simulink model "IEEE_9bus_4"  (Simulink 8.4)
settings: Solver=ode4  StartTime=0.0  StopTime=inf  FixedStep=Ts  RelTol=1e-3
PostLoadFcn:
  | Ts=25e-6;Rs=5*1.867;cs=1.4080e-004;
InitFcn:
  | Ts=25e-6;Rs=5*1.867;cs=1.4080e-004;
undefined symbols (not defined in the file): another_event_name, gcbh, my_event_name, sps_rtmsupport
libraries: spsVIMeasurementModel x36, powerlib x34, powerlib_meascontrol x18, rtlab x4, artemis x3, sps_avr x3
(part 2 of 3)

== system IEEE_9bus_4/SM_System/Bus_4 230 KV ==
  Three-Phase V-I Measurement1 : Subsystem  DialogController=POWERSYS.PowerSysDialog  LoadFcn=sps_rtmsupport('LoadFcn',gcbh);  StartFcn=sps_rtmsupport('StartFcn',gcbh);  StopFcn=sps_rtmsupport('StopFcn',gcbh);  mask(Three-Phase VI Measurement){VoltageMeasurement=phase-to-phase, SetLabelV=on, LabelV=Vabc_4, Vpu=off, VpuLL=off, CurrentMeasurement=yes, SetLabelI=on, LabelI=Iabc_4, Ipu=off, Pbase=100e6, Vbase=230e3, OutputType=Complex, PhasorSimulation=off, PSBequivalent=0}
      mask prompts: VoltageMeasurement "Voltage measurement"; SetLabelV "Use a label"; LabelV "Signal label  (use a From block to collect this signal)"; Vpu "Voltages in pu,  based on peak value of nominal phase-to-ground voltage"; VpuLL "Voltages in pu,  based on peak value of nominal phase-to-phase  voltage"; CurrentMeasurement "Current measurement"; SetLabelI "Use a label"; LabelI "Signal label  (use a From block to collect this signal)"; Ipu "Currents in pu"; Pbase "Base power ( VA 3 phase)"; Vbase "Nominal voltage used for pu measurement (Vrms phase-phase) :"; OutputType "Output signals in:"; PhasorSimulation "Phasor simulation (internal use)"; PSBequivalent "Equivalent circuit (internal use)"
      mask help:
      | Ideal three-phase voltage and current measurements.
      |
      | The block can output the voltages and currents in per unit values or in volts and amperes.
      mask init: same as IEEE_9bus_4/SM_System/Bus_1 16.5 KV
      settings: CopyFcn=sps_rtmsupport('CopyFcn',gcbh); powericon('ThreePhaseVIMeasurementCopy',gcb)  DeleteFcn=sps_rtmsupport('DeleteFcn',gcbh);  UndoDeleteFcn=sps_rtmsupport('UndoDeleteFcn',gcbh);  ModelCloseFcn=sps_rtmsupport('ModelCloseFcn',gcbh);  PreSaveFcn="sps_rtmsupport('PreSaveFcn',gcbh);  set_param(gcb,'LinkStatus','restore')"  PostSaveFcn=sps_rtmsupport('PostSaveFcn',gcbh);  NameChangeFcn=sps_rtmsupport('NameChangeFcn',gcbh);  PreCopyFcn=sps_rtmsupport('PreCopyFcn',gcbh);  OpenFcn=sps_rtmsupport('OpenFcn',gcbh, [1 2 4 5 6 7 9 -12 13]);  CloseFcn=sps_rtmsupport('CloseFcn',gcbh);  PreDeleteFcn=sps_rtmsupport('PreDeleteFcn',gcbh);
      mask Help: helpview(psbhelp)
      mask TypeOptions VoltageMeasurement: no | phase-to-ground | phase-to-phase
      mask Callback VoltageMeasurement: powericon('ThreePhaseVIMeasurementCback',gcb,'Vselector');
      mask Callback SetLabelV: powericon('ThreePhaseVIMeasurementCback',gcb,'');
      mask Callback Vpu: powericon('ThreePhaseVIMeasurementCback',gcb,'Vpu');
      mask Callback VpuLL: powericon('ThreePhaseVIMeasurementCback',gcb,'VpuLL');
      mask TypeOptions CurrentMeasurement: no | yes
      mask Callback CurrentMeasurement: powericon('ThreePhaseVIMeasurementCback',gcb,'');
      mask Callback SetLabelI: powericon('ThreePhaseVIMeasurementCback',gcb,'');
      mask Callback LabelI: powericon('ThreePhaseVIMeasurementCback',gcb,'');
      mask Callback Ipu: powericon('ThreePhaseVIMeasurementCback',gcb,'');
      mask TypeOptions OutputType: Complex | Real-Imag | Magnitude-Angle | Magnitude
  Three-Phase V-I Measurement3 : Subsystem  DialogController=POWERSYS.PowerSysDialog  LoadFcn=sps_rtmsupport('LoadFcn',gcbh);  StartFcn=sps_rtmsupport('StartFcn',gcbh);  StopFcn=sps_rtmsupport('StopFcn',gcbh);  mask(Three-Phase VI Measurement){VoltageMeasurement=phase-to-phase, SetLabelV=on, LabelV=Vabc_46, Vpu=off, VpuLL=off, CurrentMeasurement=yes, SetLabelI=on, LabelI=Iabc_46, Ipu=off, Pbase=100e6, Vbase=230e3, OutputType=Complex, PhasorSimulation=off, PSBequivalent=0}
      mask prompts: VoltageMeasurement "Voltage measurement"; SetLabelV "Use a label"; LabelV "Signal label  (use a From block to collect this signal)"; Vpu "Voltages in pu,  based on peak value of nominal phase-to-ground voltage"; VpuLL "Voltages in pu,  based on peak value of nominal phase-to-phase  voltage"; CurrentMeasurement "Current measurement"; SetLabelI "Use a label"; LabelI "Signal label  (use a From block to collect this signal)"; Ipu "Currents in pu"; Pbase "Base power ( VA 3 phase)"; Vbase "Nominal voltage used for pu measurement (Vrms phase-phase) :"; OutputType "Output signals in:"; PhasorSimulation "Phasor simulation (internal use)"; PSBequivalent "Equivalent circuit (internal use)"
      mask help:
      | Ideal three-phase voltage and current measurements.
      |
      | The block can output the voltages and currents in per unit values or in volts and amperes.
      mask init: same as IEEE_9bus_4/SM_System/Bus_1 16.5 KV
      settings: CopyFcn=sps_rtmsupport('CopyFcn',gcbh); powericon('ThreePhaseVIMeasurementCopy',gcb)  DeleteFcn=sps_rtmsupport('DeleteFcn',gcbh);  UndoDeleteFcn=sps_rtmsupport('UndoDeleteFcn',gcbh);  ModelCloseFcn=sps_rtmsupport('ModelCloseFcn',gcbh);  PreSaveFcn="sps_rtmsupport('PreSaveFcn',gcbh);  set_param(gcb,'LinkStatus','restore')"  PostSaveFcn=sps_rtmsupport('PostSaveFcn',gcbh);  NameChangeFcn=sps_rtmsupport('NameChangeFcn',gcbh);  PreCopyFcn=sps_rtmsupport('PreCopyFcn',gcbh);  OpenFcn=sps_rtmsupport('OpenFcn',gcbh, [1 2 4 5 6 7 9 -12 13]);  CloseFcn=sps_rtmsupport('CloseFcn',gcbh);  PreDeleteFcn=sps_rtmsupport('PreDeleteFcn',gcbh);
      mask Help: helpview(psbhelp)
      mask TypeOptions VoltageMeasurement: no | phase-to-ground | phase-to-phase
      mask Callback VoltageMeasurement: powericon('ThreePhaseVIMeasurementCback',gcb,'Vselector');
      mask Callback SetLabelV: powericon('ThreePhaseVIMeasurementCback',gcb,'');
      mask Callback Vpu: powericon('ThreePhaseVIMeasurementCback',gcb,'Vpu');
      mask Callback VpuLL: powericon('ThreePhaseVIMeasurementCback',gcb,'VpuLL');
      mask TypeOptions CurrentMeasurement: no | yes
      mask Callback CurrentMeasurement: powericon('ThreePhaseVIMeasurementCback',gcb,'');
      mask Callback SetLabelI: powericon('ThreePhaseVIMeasurementCback',gcb,'');
      mask Callback LabelI: powericon('ThreePhaseVIMeasurementCback',gcb,'');
      mask Callback Ipu: powericon('ThreePhaseVIMeasurementCback',gcb,'');
      mask TypeOptions OutputType: Complex | Real-Imag | Magnitude-Angle | Magnitude
  Conn7 : PMIOPort  Port=1  Side=Left
  Conn8 : PMIOPort  Port=2  Side=Left
  Conn9 : PMIOPort  Port=3  Side=Left
  Conn1 : PMIOPort  Port=4  Side=Right
  Conn2 : PMIOPort  Port=5  Side=Right
  Conn3 : PMIOPort  Port=6  Side=Right
  Conn4 : PMIOPort  Port=7  Side=Right
  Conn5 : PMIOPort  Port=8  Side=Right
  Conn6 : PMIOPort  Port=9  Side=Right
  connections:
  Three-Phase V-I Measurement3/LConn3 -- Conn9/RConn1 -- Three-Phase V-I Measurement1/LConn3
  Three-Phase V-I Measurement3/LConn2 -- Conn8/RConn1 -- Three-Phase V-I Measurement1/LConn2
  Three-Phase V-I Measurement3/LConn1 -- Conn7/RConn1 -- Three-Phase V-I Measurement1/LConn1
  Three-Phase V-I Measurement3/RConn3 -- Conn6/RConn1
  Three-Phase V-I Measurement1/RConn3 -- Conn3/RConn1
  Three-Phase V-I Measurement1/RConn1 -- Conn1/RConn1
  Three-Phase V-I Measurement1/RConn2 -- Conn2/RConn1
  Three-Phase V-I Measurement3/RConn1 -- Conn4/RConn1
  Three-Phase V-I Measurement3/RConn2 -- Conn5/RConn1

== system IEEE_9bus_4/SM_System/Bus_5 230 KV ==
  Kv : Gain  Gain=Ki  SaturateOnIntegerOverflow=on  OutDataTypeStr=Inherit: Same as input  ParamDataTypeStr=Inherit: Same as input
  Kv1 : Gain  Gain=Kv  SaturateOnIntegerOverflow=on  OutDataTypeStr=Inherit: Same as input  ParamDataTypeStr=Inherit: Same as input
  Mode I : spsVIMeasurementModel/Complex
  Mode V : spsVIMeasurementModel/Complex
  Model : spsVIMeasurementModel/VI_phase  SystemSampleTime=-1
  A : PMIOPort  Port=1  Side=Left
  B : PMIOPort  Port=2  Side=Left
  C : PMIOPort  Port=3  Side=Left
  a : PMIOPort  Port=4  Side=Right
  b : PMIOPort  Port=5  Side=Right
  c : PMIOPort  Port=6  Side=Right
  tag scope: Iabc_5=global, Vabc_5=global
  wires:
  Model/2 -> Kv/1
  Model/1 -> Kv1/1
  Kv/1 -> Mode I/1
  Kv1/1 -> Mode V/1
  Mode I/1 -> [Iabc_5]
  Mode V/1 -> [Vabc_5]
  connections:
  Model/RConn3 -- c/RConn1
  Model/RConn1 -- a/RConn1
  Model/RConn2 -- b/RConn1
  Model/LConn3 -- C/RConn1
  Model/LConn1 -- A/RConn1
  Model/LConn2 -- B/RConn1

== system IEEE_9bus_4/SM_System/Bus_6 230 KV ==
  Kv : Gain  Gain=Ki  SaturateOnIntegerOverflow=on  OutDataTypeStr=Inherit: Same as input  ParamDataTypeStr=Inherit: Same as input
  Kv1 : Gain  Gain=Kv  SaturateOnIntegerOverflow=on  OutDataTypeStr=Inherit: Same as input  ParamDataTypeStr=Inherit: Same as input
  Mode I : spsVIMeasurementModel/Complex
  Mode V : spsVIMeasurementModel/Complex
  Model : spsVIMeasurementModel/VI_phase  SystemSampleTime=-1
  A : PMIOPort  Port=1  Side=Left
  B : PMIOPort  Port=2  Side=Left
  C : PMIOPort  Port=3  Side=Left
  a : PMIOPort  Port=4  Side=Right
  b : PMIOPort  Port=5  Side=Right
  c : PMIOPort  Port=6  Side=Right
  tag scope: Iabc_6=global, Vabc_6=global
  wires:
  Model/2 -> Kv/1
  Model/1 -> Kv1/1
  Kv/1 -> Mode I/1
  Kv1/1 -> Mode V/1
  Mode I/1 -> [Iabc_6]
  Mode V/1 -> [Vabc_6]
  connections:
  Model/RConn3 -- c/RConn1
  Model/RConn1 -- a/RConn1
  Model/RConn2 -- b/RConn1
  Model/LConn3 -- C/RConn1
  Model/LConn1 -- A/RConn1
  Model/LConn2 -- B/RConn1

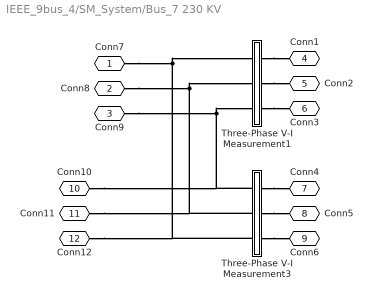
== system IEEE_9bus_4/SM_System/Bus_7 230 KV ==
  Three-Phase V-I Measurement1 : Subsystem  DialogController=POWERSYS.PowerSysDialog  LoadFcn=sps_rtmsupport('LoadFcn',gcbh);  StartFcn=sps_rtmsupport('StartFcn',gcbh);  StopFcn=sps_rtmsupport('StopFcn',gcbh);  mask(Three-Phase VI Measurement){VoltageMeasurement=phase-to-phase, SetLabelV=on, LabelV=Vabc_7, Vpu=off, VpuLL=off, CurrentMeasurement=yes, SetLabelI=on, LabelI=Iabc_7, Ipu=off, Pbase=100e6, Vbase=230e3, OutputType=Complex, PhasorSimulation=off, PSBequivalent=0}
      mask prompts: VoltageMeasurement "Voltage measurement"; SetLabelV "Use a label"; LabelV "Signal label  (use a From block to collect this signal)"; Vpu "Voltages in pu,  based on peak value of nominal phase-to-ground voltage"; VpuLL "Voltages in pu,  based on peak value of nominal phase-to-phase  voltage"; CurrentMeasurement "Current measurement"; SetLabelI "Use a label"; LabelI "Signal label  (use a From block to collect this signal)"; Ipu "Currents in pu"; Pbase "Base power ( VA 3 phase)"; Vbase "Nominal voltage used for pu measurement (Vrms phase-phase) :"; OutputType "Output signals in:"; PhasorSimulation "Phasor simulation (internal use)"; PSBequivalent "Equivalent circuit (internal use)"
      mask help:
      | Ideal three-phase voltage and current measurements.
      |
      | The block can output the voltages and currents in per unit values or in volts and amperes.
      mask init: same as IEEE_9bus_4/SM_System/Bus_1 16.5 KV
      settings: CopyFcn=sps_rtmsupport('CopyFcn',gcbh); powericon('ThreePhaseVIMeasurementCopy',gcb)  DeleteFcn=sps_rtmsupport('DeleteFcn',gcbh);  UndoDeleteFcn=sps_rtmsupport('UndoDeleteFcn',gcbh);  ModelCloseFcn=sps_rtmsupport('ModelCloseFcn',gcbh);  PreSaveFcn="sps_rtmsupport('PreSaveFcn',gcbh);  set_param(gcb,'LinkStatus','restore')"  PostSaveFcn=sps_rtmsupport('PostSaveFcn',gcbh);  NameChangeFcn=sps_rtmsupport('NameChangeFcn',gcbh);  PreCopyFcn=sps_rtmsupport('PreCopyFcn',gcbh);  OpenFcn=sps_rtmsupport('OpenFcn',gcbh, [1 2 4 5 6 7 9 -12 13]);  CloseFcn=sps_rtmsupport('CloseFcn',gcbh);  PreDeleteFcn=sps_rtmsupport('PreDeleteFcn',gcbh);
      mask Help: helpview(psbhelp)
      mask TypeOptions VoltageMeasurement: no | phase-to-ground | phase-to-phase
      mask Callback VoltageMeasurement: powericon('ThreePhaseVIMeasurementCback',gcb,'Vselector');
      mask Callback SetLabelV: powericon('ThreePhaseVIMeasurementCback',gcb,'');
      mask Callback Vpu: powericon('ThreePhaseVIMeasurementCback',gcb,'Vpu');
      mask Callback VpuLL: powericon('ThreePhaseVIMeasurementCback',gcb,'VpuLL');
      mask TypeOptions CurrentMeasurement: no | yes
      mask Callback CurrentMeasurement: powericon('ThreePhaseVIMeasurementCback',gcb,'');
      mask Callback SetLabelI: powericon('ThreePhaseVIMeasurementCback',gcb,'');
      mask Callback LabelI: powericon('ThreePhaseVIMeasurementCback',gcb,'');
      mask Callback Ipu: powericon('ThreePhaseVIMeasurementCback',gcb,'');
      mask TypeOptions OutputType: Complex | Real-Imag | Magnitude-Angle | Magnitude
  Three-Phase V-I Measurement3 : Subsystem  DialogController=POWERSYS.PowerSysDialog  LoadFcn=sps_rtmsupport('LoadFcn',gcbh);  StartFcn=sps_rtmsupport('StartFcn',gcbh);  StopFcn=sps_rtmsupport('StopFcn',gcbh);  mask(Three-Phase VI Measurement){VoltageMeasurement=phase-to-phase, SetLabelV=on, LabelV=Vabc, Vpu=off, VpuLL=off, CurrentMeasurement=yes, SetLabelI=on, LabelI=Iab, Ipu=off, Pbase=100e6, Vbase=230e3, OutputType=Complex, PhasorSimulation=off, PSBequivalent=0}
      mask prompts: VoltageMeasurement "Voltage measurement"; SetLabelV "Use a label"; LabelV "Signal label  (use a From block to collect this signal)"; Vpu "Voltages in pu,  based on peak value of nominal phase-to-ground voltage"; VpuLL "Voltages in pu,  based on peak value of nominal phase-to-phase  voltage"; CurrentMeasurement "Current measurement"; SetLabelI "Use a label"; LabelI "Signal label  (use a From block to collect this signal)"; Ipu "Currents in pu"; Pbase "Base power ( VA 3 phase)"; Vbase "Nominal voltage used for pu measurement (Vrms phase-phase) :"; OutputType "Output signals in:"; PhasorSimulation "Phasor simulation (internal use)"; PSBequivalent "Equivalent circuit (internal use)"
      mask help:
      | Ideal three-phase voltage and current measurements.
      |
      | The block can output the voltages and currents in per unit values or in volts and amperes.
      mask init: same as IEEE_9bus_4/SM_System/Bus_1 16.5 KV
      settings: CopyFcn=sps_rtmsupport('CopyFcn',gcbh); powericon('ThreePhaseVIMeasurementCopy',gcb)  DeleteFcn=sps_rtmsupport('DeleteFcn',gcbh);  UndoDeleteFcn=sps_rtmsupport('UndoDeleteFcn',gcbh);  ModelCloseFcn=sps_rtmsupport('ModelCloseFcn',gcbh);  PreSaveFcn="sps_rtmsupport('PreSaveFcn',gcbh);  set_param(gcb,'LinkStatus','restore')"  PostSaveFcn=sps_rtmsupport('PostSaveFcn',gcbh);  NameChangeFcn=sps_rtmsupport('NameChangeFcn',gcbh);  PreCopyFcn=sps_rtmsupport('PreCopyFcn',gcbh);  OpenFcn=sps_rtmsupport('OpenFcn',gcbh, [1 2 4 5 6 7 9 -12 13]);  CloseFcn=sps_rtmsupport('CloseFcn',gcbh);  PreDeleteFcn=sps_rtmsupport('PreDeleteFcn',gcbh);
      mask Help: helpview(psbhelp)
      mask TypeOptions VoltageMeasurement: no | phase-to-ground | phase-to-phase
      mask Callback VoltageMeasurement: powericon('ThreePhaseVIMeasurementCback',gcb,'Vselector');
      mask Callback SetLabelV: powericon('ThreePhaseVIMeasurementCback',gcb,'');
      mask Callback Vpu: powericon('ThreePhaseVIMeasurementCback',gcb,'Vpu');
      mask Callback VpuLL: powericon('ThreePhaseVIMeasurementCback',gcb,'VpuLL');
      mask TypeOptions CurrentMeasurement: no | yes
      mask Callback CurrentMeasurement: powericon('ThreePhaseVIMeasurementCback',gcb,'');
      mask Callback SetLabelI: powericon('ThreePhaseVIMeasurementCback',gcb,'');
      mask Callback LabelI: powericon('ThreePhaseVIMeasurementCback',gcb,'');
      mask Callback Ipu: powericon('ThreePhaseVIMeasurementCback',gcb,'');
      mask TypeOptions OutputType: Complex | Real-Imag | Magnitude-Angle | Magnitude
  Conn7 : PMIOPort  Port=1  Side=Left
  Conn8 : PMIOPort  Port=2  Side=Left
  Conn9 : PMIOPort  Port=3  Side=Left
  Conn1 : PMIOPort  Port=4  Side=Right
  Conn2 : PMIOPort  Port=5  Side=Right
  Conn3 : PMIOPort  Port=6  Side=Right
  Conn4 : PMIOPort  Port=7  Side=Right
  Conn5 : PMIOPort  Port=8  Side=Right
  Conn6 : PMIOPort  Port=9  Side=Right
  Conn10 : PMIOPort  Port=10  Side=Left
  Conn11 : PMIOPort  Port=11  Side=Left
  Conn12 : PMIOPort  Port=12  Side=Left
  connections:
  Three-Phase V-I Measurement3/RConn2 -- Conn5/RConn1
  Three-Phase V-I Measurement3/RConn1 -- Conn4/RConn1
  Three-Phase V-I Measurement1/RConn2 -- Conn2/RConn1
  Three-Phase V-I Measurement1/RConn1 -- Conn1/RConn1
  Three-Phase V-I Measurement1/RConn3 -- Conn3/RConn1
  Three-Phase V-I Measurement3/RConn3 -- Conn6/RConn1
  Conn7/RConn1 -- Three-Phase V-I Measurement3/LConn3 -- Conn12/RConn1 -- Three-Phase V-I Measurement1/LConn1
  Conn8/RConn1 -- Three-Phase V-I Measurement3/LConn2 -- Conn11/RConn1 -- Three-Phase V-I Measurement1/LConn2
  Conn9/RConn1 -- Conn10/RConn1 -- Three-Phase V-I Measurement3/LConn1 -- Three-Phase V-I Measurement1/LConn3

== system IEEE_9bus_4/SM_System/Bus_8 230 KV ==
  Kv : Gain  Gain=Ki  SaturateOnIntegerOverflow=on  OutDataTypeStr=Inherit: Same as input  ParamDataTypeStr=Inherit: Same as input
  Kv1 : Gain  Gain=Kv  SaturateOnIntegerOverflow=on  OutDataTypeStr=Inherit: Same as input  ParamDataTypeStr=Inherit: Same as input
  Mode I : spsVIMeasurementModel/Complex
  Mode V : spsVIMeasurementModel/Complex
  Model : spsVIMeasurementModel/VI_phase  SystemSampleTime=-1
  A : PMIOPort  Port=1  Side=Left
  B : PMIOPort  Port=2  Side=Left
  C : PMIOPort  Port=3  Side=Left
  a : PMIOPort  Port=4  Side=Right
  b : PMIOPort  Port=5  Side=Right
  c : PMIOPort  Port=6  Side=Right
  tag scope: Iabc_8=global, Vabc_8=global
  wires:
  Model/2 -> Kv/1
  Model/1 -> Kv1/1
  Kv/1 -> Mode I/1
  Kv1/1 -> Mode V/1
  Mode I/1 -> [Iabc_8]
  Mode V/1 -> [Vabc_8]
  connections:
  Model/RConn3 -- c/RConn1
  Model/RConn1 -- a/RConn1
  Model/RConn2 -- b/RConn1
  Model/LConn3 -- C/RConn1
  Model/LConn1 -- A/RConn1
  Model/LConn2 -- B/RConn1

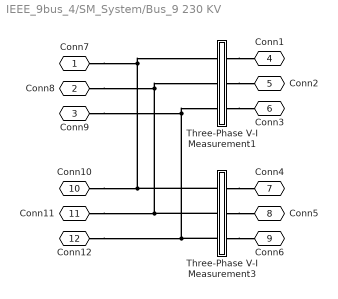
== system IEEE_9bus_4/SM_System/Bus_9 230 KV ==
  Three-Phase V-I Measurement1 : Subsystem  DialogController=POWERSYS.PowerSysDialog  LoadFcn=sps_rtmsupport('LoadFcn',gcbh);  StartFcn=sps_rtmsupport('StartFcn',gcbh);  StopFcn=sps_rtmsupport('StopFcn',gcbh);  mask(Three-Phase VI Measurement){VoltageMeasurement=phase-to-phase, SetLabelV=on, LabelV=Vabc_9, Vpu=off, VpuLL=off, CurrentMeasurement=yes, SetLabelI=on, LabelI=Iabc_9, Ipu=off, Pbase=100e6, Vbase=230e3, OutputType=Complex, PhasorSimulation=off, PSBequivalent=0}
      mask prompts: VoltageMeasurement "Voltage measurement"; SetLabelV "Use a label"; LabelV "Signal label  (use a From block to collect this signal)"; Vpu "Voltages in pu,  based on peak value of nominal phase-to-ground voltage"; VpuLL "Voltages in pu,  based on peak value of nominal phase-to-phase  voltage"; CurrentMeasurement "Current measurement"; SetLabelI "Use a label"; LabelI "Signal label  (use a From block to collect this signal)"; Ipu "Currents in pu"; Pbase "Base power ( VA 3 phase)"; Vbase "Nominal voltage used for pu measurement (Vrms phase-phase) :"; OutputType "Output signals in:"; PhasorSimulation "Phasor simulation (internal use)"; PSBequivalent "Equivalent circuit (internal use)"
      mask help:
      | Ideal three-phase voltage and current measurements.
      |
      | The block can output the voltages and currents in per unit values or in volts and amperes.
      mask init: same as IEEE_9bus_4/SM_System/Bus_1 16.5 KV
      settings: CopyFcn=sps_rtmsupport('CopyFcn',gcbh); powericon('ThreePhaseVIMeasurementCopy',gcb)  DeleteFcn=sps_rtmsupport('DeleteFcn',gcbh);  UndoDeleteFcn=sps_rtmsupport('UndoDeleteFcn',gcbh);  ModelCloseFcn=sps_rtmsupport('ModelCloseFcn',gcbh);  PreSaveFcn="sps_rtmsupport('PreSaveFcn',gcbh);  set_param(gcb,'LinkStatus','restore')"  PostSaveFcn=sps_rtmsupport('PostSaveFcn',gcbh);  NameChangeFcn=sps_rtmsupport('NameChangeFcn',gcbh);  PreCopyFcn=sps_rtmsupport('PreCopyFcn',gcbh);  OpenFcn=sps_rtmsupport('OpenFcn',gcbh, [1 2 4 5 6 7 9 -12 13]);  CloseFcn=sps_rtmsupport('CloseFcn',gcbh);  PreDeleteFcn=sps_rtmsupport('PreDeleteFcn',gcbh);
      mask Help: helpview(psbhelp)
      mask TypeOptions VoltageMeasurement: no | phase-to-ground | phase-to-phase
      mask Callback VoltageMeasurement: powericon('ThreePhaseVIMeasurementCback',gcb,'Vselector');
      mask Callback SetLabelV: powericon('ThreePhaseVIMeasurementCback',gcb,'');
      mask Callback Vpu: powericon('ThreePhaseVIMeasurementCback',gcb,'Vpu');
      mask Callback VpuLL: powericon('ThreePhaseVIMeasurementCback',gcb,'VpuLL');
      mask TypeOptions CurrentMeasurement: no | yes
      mask Callback CurrentMeasurement: powericon('ThreePhaseVIMeasurementCback',gcb,'');
      mask Callback SetLabelI: powericon('ThreePhaseVIMeasurementCback',gcb,'');
      mask Callback LabelI: powericon('ThreePhaseVIMeasurementCback',gcb,'');
      mask Callback Ipu: powericon('ThreePhaseVIMeasurementCback',gcb,'');
      mask TypeOptions OutputType: Complex | Real-Imag | Magnitude-Angle | Magnitude
  Three-Phase V-I Measurement3 : Subsystem  DialogController=POWERSYS.PowerSysDialog  LoadFcn=sps_rtmsupport('LoadFcn',gcbh);  StartFcn=sps_rtmsupport('StartFcn',gcbh);  StopFcn=sps_rtmsupport('StopFcn',gcbh);  mask(Three-Phase VI Measurement){VoltageMeasurement=phase-to-phase, SetLabelV=on, LabelV=Vabc_10, Vpu=off, VpuLL=off, CurrentMeasurement=yes, SetLabelI=on, LabelI=Iabc, Ipu=off, Pbase=100e6, Vbase=230e3, OutputType=Complex, PhasorSimulation=off, PSBequivalent=0}
      mask prompts: VoltageMeasurement "Voltage measurement"; SetLabelV "Use a label"; LabelV "Signal label  (use a From block to collect this signal)"; Vpu "Voltages in pu,  based on peak value of nominal phase-to-ground voltage"; VpuLL "Voltages in pu,  based on peak value of nominal phase-to-phase  voltage"; CurrentMeasurement "Current measurement"; SetLabelI "Use a label"; LabelI "Signal label  (use a From block to collect this signal)"; Ipu "Currents in pu"; Pbase "Base power ( VA 3 phase)"; Vbase "Nominal voltage used for pu measurement (Vrms phase-phase) :"; OutputType "Output signals in:"; PhasorSimulation "Phasor simulation (internal use)"; PSBequivalent "Equivalent circuit (internal use)"
      mask help:
      | Ideal three-phase voltage and current measurements.
      |
      | The block can output the voltages and currents in per unit values or in volts and amperes.
      mask init: same as IEEE_9bus_4/SM_System/Bus_1 16.5 KV
      settings: CopyFcn=sps_rtmsupport('CopyFcn',gcbh); powericon('ThreePhaseVIMeasurementCopy',gcb)  DeleteFcn=sps_rtmsupport('DeleteFcn',gcbh);  UndoDeleteFcn=sps_rtmsupport('UndoDeleteFcn',gcbh);  ModelCloseFcn=sps_rtmsupport('ModelCloseFcn',gcbh);  PreSaveFcn="sps_rtmsupport('PreSaveFcn',gcbh);  set_param(gcb,'LinkStatus','restore')"  PostSaveFcn=sps_rtmsupport('PostSaveFcn',gcbh);  NameChangeFcn=sps_rtmsupport('NameChangeFcn',gcbh);  PreCopyFcn=sps_rtmsupport('PreCopyFcn',gcbh);  OpenFcn=sps_rtmsupport('OpenFcn',gcbh, [1 2 4 5 6 7 9 -12 13]);  CloseFcn=sps_rtmsupport('CloseFcn',gcbh);  PreDeleteFcn=sps_rtmsupport('PreDeleteFcn',gcbh);
      mask Help: helpview(psbhelp)
      mask TypeOptions VoltageMeasurement: no | phase-to-ground | phase-to-phase
      mask Callback VoltageMeasurement: powericon('ThreePhaseVIMeasurementCback',gcb,'Vselector');
      mask Callback SetLabelV: powericon('ThreePhaseVIMeasurementCback',gcb,'');
      mask Callback Vpu: powericon('ThreePhaseVIMeasurementCback',gcb,'Vpu');
      mask Callback VpuLL: powericon('ThreePhaseVIMeasurementCback',gcb,'VpuLL');
      mask TypeOptions CurrentMeasurement: no | yes
      mask Callback CurrentMeasurement: powericon('ThreePhaseVIMeasurementCback',gcb,'');
      mask Callback SetLabelI: powericon('ThreePhaseVIMeasurementCback',gcb,'');
      mask Callback LabelI: powericon('ThreePhaseVIMeasurementCback',gcb,'');
      mask Callback Ipu: powericon('ThreePhaseVIMeasurementCback',gcb,'');
      mask TypeOptions OutputType: Complex | Real-Imag | Magnitude-Angle | Magnitude
  Conn7 : PMIOPort  Port=1  Side=Left
  Conn8 : PMIOPort  Port=2  Side=Left
  Conn9 : PMIOPort  Port=3  Side=Left
  Conn1 : PMIOPort  Port=4  Side=Right
  Conn2 : PMIOPort  Port=5  Side=Right
  Conn3 : PMIOPort  Port=6  Side=Right
  Conn4 : PMIOPort  Port=7  Side=Right
  Conn5 : PMIOPort  Port=8  Side=Right
  Conn6 : PMIOPort  Port=9  Side=Right
  Conn10 : PMIOPort  Port=10  Side=Left
  Conn11 : PMIOPort  Port=11  Side=Left
  Conn12 : PMIOPort  Port=12  Side=Left
  connections:
  Conn12/RConn1 -- Three-Phase V-I Measurement3/LConn3 -- Conn9/RConn1 -- Three-Phase V-I Measurement1/LConn3
  Conn11/RConn1 -- Three-Phase V-I Measurement3/LConn2 -- Conn8/RConn1 -- Three-Phase V-I Measurement1/LConn2
  Conn10/RConn1 -- Three-Phase V-I Measurement3/LConn1 -- Conn7/RConn1 -- Three-Phase V-I Measurement1/LConn1
  Three-Phase V-I Measurement3/RConn3 -- Conn6/RConn1
  Three-Phase V-I Measurement1/RConn3 -- Conn3/RConn1
  Three-Phase V-I Measurement1/RConn1 -- Conn1/RConn1
  Three-Phase V-I Measurement1/RConn2 -- Conn2/RConn1
  Three-Phase V-I Measurement3/RConn1 -- Conn4/RConn1
  Three-Phase V-I Measurement3/RConn2 -- Conn5/RConn1

== system IEEE_9bus_4/SM_System/Fault_Gen ==
  In1 : Inport
  Constant1 : Constant  Value=[0 0]  SampleTime=-1
  Demux4 : Demux  Outputs=[1 3 3 1 1 1 1]
  Sine Wave : Sin  Frequency=2*pi*60  SampleTime=Ts
  faultgen : Subsystem
  Fault : Outport
  Pert : Outport  Port=2
  TTigger : Outport  Port=3
  tag scope: L1=global, L2=global, L3=global, fault_type=global
  wires:
  Sine Wave/1 -> faultgen/6(pulse)
  Constant1/1 -> faultgen/5(pert_set)
  Demux4/1 -> faultgen/1(Tacq)
  Demux4/2 -> faultgen/2(Tst_set)
  Demux4/3 -> faultgen/3(Tdr_set)
  Demux4/4 -> faultgen/4(faultype), [fault_type]
  Demux4/5 -> [L1]
  faultgen/1(fault) -> Fault/1
  In1/1 -> Demux4/1
  faultgen/2(pertb) -> Pert/1
  faultgen/3(trig) -> TTigger/1
  Demux4/6 -> [L2]
  Demux4/7 -> [L3]

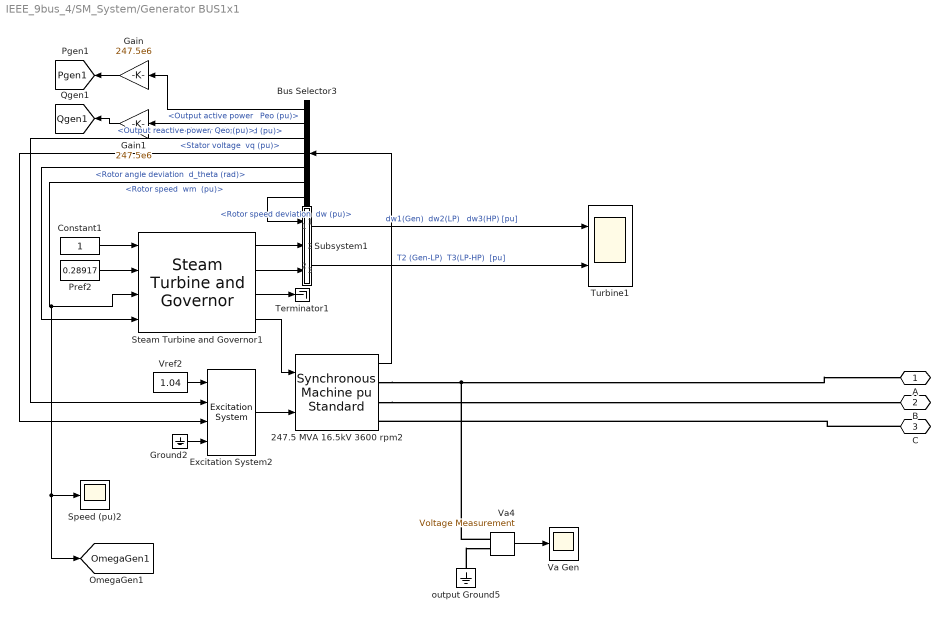
== system IEEE_9bus_4/SM_System/Generator BUS1x1 ==
  " Speed (pu)2" : Scope
      settings: TickLabels=on  TimeRange=100  YMin=0.995  YMax=1  SaveName=Gen1Freq
  247.5 MVA 16.5kV 3600 rpm2 : powerlib/Machines/Synchronous Machine pu Standard  PresetModel=No  MechanicalLoad=Mechanical power Pm  ShowDetailedParameters=on  RotorType=Round  Units=per unit standard parameters  MeasurementBus=off  NominalParameters="[ 247.5e6  16.5e3   60 ]"  Reactances1=[ 0.36135, 0.15048, 0.12375, 0.2475, 0.2398275, 0.12375, 0.08316 ]  Reactances2="[ 1.305, 0.296, 0.252, 0.474,  0.243,  0.18 ]"  dAxisTimeConstants=Open-circuit  qAxisTimeConstants=Open-circuit  TimeConstants1="[ 4.4849  0.0681  0.1  ]"  TimeConstants2="[ 8.96, 0.05,  0.31, 0.05 ]"  TimeConstants3="[  4.49  0.0681  0.0513  ]"  TimeConstants4=[ 8.0, 0.03, 0.3371, 0.0295 ]  TimeConstants5=[ 1.01, 0.053, 0.1 ]  TimeConstants6=[ 1.3201, 0.023, 1.0, 0.07 ]  TimeConstants7="[  1.01  0.053  0.051266  ]"  TimeConstants8=[ 1.3201, 0.0231, 0.3371, 0.0295 ]  StatorResistance=0.000125  Mechanical="[ 23.64  0 1 ]"  PolePairs=1  InitialConditions=[0 -86.3058 0.296671 0.296671 0.296671 -20.4087 -140.409 99.5913 1.08165]  SetSaturation=off  Saturation=[0.6404,0.7127,0.8441,0.9214,0.9956,1.082,1.19,1.316,1.457;0.7,0.7698,0.8872,0.9466,0.9969,1.046,1.1,1.151,1.201]  LoadFlowParameters=[2 71600000 0 0 0]  TsPowergui=0  TsBlock=-1  IterativeModel=Trapezoidal non iterative  BusType=swing  Pref=0  Qref=0  Qmin=-Inf  Qmax=Inf  PLF=0  QLF=0
  Bus Selector3 : BusSelector  OutputSignals="Output active power   Peo (pu),Output reactive power  Qeo (pu),dq0 components.Stator voltage  vd (pu),dq0 components.Stator voltage  vq (pu),Mechanical.Rotor angle deviation  d_theta (rad),Mechanical.Rotor speed  wm  (pu),Mechanical.Rotor speed deviation  dw (pu)"
  Constant1 : Constant
  Excitation System2 : sps_avr/Excitation System  tr=20e-3  reg=[ 200, 0.02 ]  exc=[ 1, 0 ]  tgr=[ 12.0, 1.0 ]  damp=[ 0.03, 1.0 ]  sat=[ 0, 0 ]  lim=[ -10.0, 10.0, 0 ]  v0=[1.04 1.0817]
  Gain : Gain  Gain=247.5e6
  Gain1 : Gain  Gain=247.5e6
  Ground2 : Ground
  Pref2 : Constant  Value=0.28917
  Steam Turbine and Governor1 : powerlib/Machines/Steam Turbine and Governor  gentype=Tandem-compound (single mass)  reg1="[ 1  0.05    0 ]"  reg2="[ 0.001  0.1 ]"  reg3="[ -10.0 0.1   0.1 1.0 ]"  N=3600  turb1="[ 0.12  0.13  10.0   0.32   ]"  turb2="[ 0.48   0.25   0  0.27 ]"  HA="[  1.5498   0.24894  0  0 ]"  KA="[  83.47  42.702  0  0 ]"  DA="[  0.3104  0.05  0  0 ]*8"  ini1=0.28918  ini2=[1.88924e-008,-120.067]
  Subsystem1 : Subsystem
  Terminator1 : Terminator
  Turbine1 : Scope  NumInputPorts=2
      settings: TimeRange=0.5  YMin=0~-1  YMax=3e+09~1  SaveName=ScopeData2
  Va Gen : Scope
      settings: TickLabels=on  TimeRange=2  YMin=-15000  YMax=15000  SaveName=vf4
  Va4 : powerlib/Measurements/Voltage Measurement  Tag=PoWeRsYsTeMmEaSuReMeNt  PhasorSimulation=off  OutputType=Magnitude  PSBequivalent=0
  Vref2 : Constant  Value=1.04
  output Ground5 : powerlib/Elements/Ground  LConnTagsString=a
  A : PMIOPort  Port=1  Side=Right
  B : PMIOPort  Port=2  Side=Right
  C : PMIOPort  Port=3  Side=Right
  tag scope: OmegaGen1=global, Pgen1=global, Qgen1=global
  wires:
  Constant1/1 -> Steam Turbine and Governor1/1
  Bus Selector3/5 -> Steam Turbine and Governor1/4  "<Rotor angle deviation  d_theta (rad)>"
  Subsystem1/2(T_23) -> Turbine1/2  "T2 (Gen-LP)  T3(LP-HP)  [pu]"
  Steam Turbine and Governor1/3 -> Terminator1/1
  Bus Selector3/7 -> Subsystem1/1(In1)  "<Rotor speed deviation  dw (pu)>"
  Vref2/1 -> Excitation System2/1
  Pref2/1 -> Steam Turbine and Governor1/2
  Steam Turbine and Governor1/1 -> Subsystem1/2(In2)
  Subsystem1/1(dw_123) -> Turbine1/1  "dw1(Gen)  dw2(LP)   dw3(HP) [pu]"
  Steam Turbine and Governor1/4 -> 247.5 MVA 16.5kV 3600 rpm2/1
  Steam Turbine and Governor1/2 -> Subsystem1/3(In3)
  Bus Selector3/6 -> [OmegaGen1], " Speed (pu)2"/1, Steam Turbine and Governor1/3  "<Rotor speed  wm  (pu)>"
  247.5 MVA 16.5kV 3600 rpm2/1 -> Bus Selector3/1
  Ground2/1 -> Excitation System2/4
  Bus Selector3/4 -> Excitation System2/3  "<Stator voltage  vq (pu)>"
  Bus Selector3/3 -> Excitation System2/2  "<Stator voltage  vd (pu)>"
  Excitation System2/1 -> 247.5 MVA 16.5kV 3600 rpm2/2
  Va4/1 -> Va Gen/1
  Bus Selector3/1 -> Gain/1  "<Output active power   Peo (pu)>"
  Bus Selector3/2 -> Gain1/1  "<Output reactive power  Qeo (pu)>"
  Gain/1 -> [Pgen1]
  Gain1/1 -> [Qgen1]
  connections:
  output Ground5/LConn1 -- Va4/LConn2
  C/RConn1 -- 247.5 MVA 16.5kV 3600 rpm2/RConn3
  247.5 MVA 16.5kV 3600 rpm2/RConn2 -- B/RConn1
  Va4/LConn1 -- 247.5 MVA 16.5kV 3600 rpm2/RConn1 -- A/RConn1

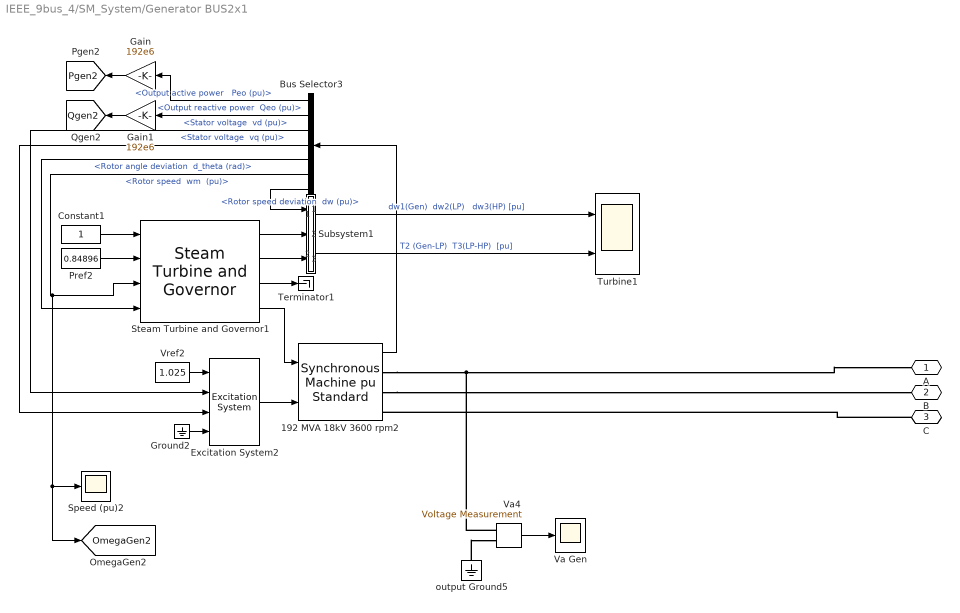
== system IEEE_9bus_4/SM_System/Generator BUS2x1 ==
  " Speed (pu)2" : Scope
      settings: TickLabels=on  TimeRange=150  YMin=0.995  YMax=1  SaveName=Pm2
  192 MVA 18kV 3600 rpm2 : powerlib/Machines/Synchronous Machine pu Standard  PresetModel=No  MechanicalLoad=Mechanical power Pm  ShowDetailedParameters=on  RotorType=Round  Units=per unit standard parameters  MeasurementBus=off  NominalParameters="[ 192e6  18e3   60 ]"  Reactances1=[ 1.719936, 0.230016, 0.1632, 1.65984, 0.378048, 0.2304, 0.10002 ]  Reactances2="[ 1.305, 0.296, 0.252, 0.474,  0.243,  0.18 ]"  dAxisTimeConstants=Open-circuit  qAxisTimeConstants=Open-circuit  TimeConstants1="[ 4.4849  0.0681  0.1  ]"  TimeConstants2="[ 6.0, 0.05,  0.535, 0.05 ]"  TimeConstants3="[  4.49  0.0681  0.0513  ]"  TimeConstants4=[ 8.0, 0.03, 0.3371, 0.0295 ]  TimeConstants5=[ 1.01, 0.053, 0.1 ]  TimeConstants6=[ 1.3201, 0.023, 1.0, 0.07 ]  TimeConstants7="[  1.01  0.053  0.051266  ]"  TimeConstants8=[ 1.3201, 0.0231, 0.3371, 0.0295 ]  StatorResistance=0.000125  Mechanical="[ 6.4  0 1 ]"  PolePairs=1  InitialConditions=[0 -28.9349 0.828916 0.828916 0.828916 6.92884 -113.071 126.929 1.78871]  SetSaturation=off  Saturation=[0.6404,0.7127,0.8441,0.9214,0.9956,1.082,1.19,1.316,1.457;0.7,0.7698,0.8872,0.9466,0.9969,1.046,1.1,1.151,1.201]  LoadFlowParameters=[1 163000000 0 0 0]  TsPowergui=0  TsBlock=-1  IterativeModel=Trapezoidal non iterative  BusType=PV  Pref=163e6  Qref=0  Qmin=-Inf  Qmax=Inf  PLF=0  QLF=0
  Bus Selector3 : BusSelector  OutputSignals="Output active power   Peo (pu),Output reactive power  Qeo (pu),dq0 components.Stator voltage  vd (pu),dq0 components.Stator voltage  vq (pu),Mechanical.Rotor angle deviation  d_theta (rad),Mechanical.Rotor speed  wm  (pu),Mechanical.Rotor speed deviation  dw (pu)"
  Constant1 : Constant
  Excitation System2 : sps_avr/Excitation System  tr=20e-3  reg=[ 200, 0.02 ]  exc=[ 1, 0 ]  tgr=[ 12.0, 1.0 ]  damp=[ 0.03, 1.0 ]  sat=[ 0, 0 ]  lim=[ -10.0, 10.0, 0 ]  v0=[1.025 1.7887]
  Gain : Gain  Gain=192e6
  Gain1 : Gain  Gain=192e6
  Ground2 : Ground
  Pref2 : Constant  Value=0.84896
  Steam Turbine and Governor1 : powerlib/Machines/Steam Turbine and Governor  gentype=Tandem-compound (single mass)  reg1="[ 1  0.05    0 ]"  reg2="[ 0.001  0.1 ]"  reg3="[ -10.0 0.1   0.1 1.0 ]"  N=3600  turb1="[ 0.12  0.13  10.0   0.32   ]"  turb2="[ 0.48   0.25   0  0.27 ]"  HA="[  1.5498   0.24894  0  0 ]"  KA="[  83.47  42.702  0  0 ]"  DA="[  0.3104  0.05  0  0 ]*8"  ini1=0.84904  ini2=[1.88924e-008,-120.067]
  Subsystem1 : Subsystem
  Terminator1 : Terminator
  Turbine1 : Scope  NumInputPorts=2
      settings: TimeRange=0.5  YMin=-0.03~-5  YMax=0.03~5  SaveName=ScopeData2
  Va Gen : Scope
      settings: TickLabels=on  TimeRange=150  YMin=-20000  YMax=20000  SaveName=vf4
  Va4 : powerlib/Measurements/Voltage Measurement  Tag=PoWeRsYsTeMmEaSuReMeNt  PhasorSimulation=off  OutputType=Magnitude  PSBequivalent=0
  Vref2 : Constant  Value=1.025
  output Ground5 : powerlib/Elements/Ground  LConnTagsString=a
  A : PMIOPort  Port=1  Side=Right
  B : PMIOPort  Port=2  Side=Right
  C : PMIOPort  Port=3  Side=Right
  tag scope: OmegaGen2=global, Pgen2=global, Qgen2=global
  wires:
  Constant1/1 -> Steam Turbine and Governor1/1
  Bus Selector3/5 -> Steam Turbine and Governor1/4  "<Rotor angle deviation  d_theta (rad)>"
  Subsystem1/2(T_23) -> Turbine1/2  "T2 (Gen-LP)  T3(LP-HP)  [pu]"
  Steam Turbine and Governor1/3 -> Terminator1/1
  Bus Selector3/7 -> Subsystem1/1(In1)  "<Rotor speed deviation  dw (pu)>"
  Vref2/1 -> Excitation System2/1
  Pref2/1 -> Steam Turbine and Governor1/2
  Steam Turbine and Governor1/1 -> Subsystem1/2(In2)
  Subsystem1/1(dw_123) -> Turbine1/1  "dw1(Gen)  dw2(LP)   dw3(HP) [pu]"
  Steam Turbine and Governor1/4 -> 192 MVA 18kV 3600 rpm2/1
  Steam Turbine and Governor1/2 -> Subsystem1/3(In3)
  Bus Selector3/6 -> [OmegaGen2], " Speed (pu)2"/1, Steam Turbine and Governor1/3  "<Rotor speed  wm  (pu)>"
  192 MVA 18kV 3600 rpm2/1 -> Bus Selector3/1
  Ground2/1 -> Excitation System2/4
  Bus Selector3/4 -> Excitation System2/3  "<Stator voltage  vq (pu)>"
  Bus Selector3/3 -> Excitation System2/2  "<Stator voltage  vd (pu)>"
  Excitation System2/1 -> 192 MVA 18kV 3600 rpm2/2
  Va4/1 -> Va Gen/1
  Bus Selector3/2 -> Gain1/1  "<Output reactive power  Qeo (pu)>"
  Bus Selector3/1 -> Gain/1  "<Output active power   Peo (pu)>"
  Gain/1 -> [Pgen2]
  Gain1/1 -> [Qgen2]
  connections:
  output Ground5/LConn1 -- Va4/LConn2
  C/RConn1 -- 192 MVA 18kV 3600 rpm2/RConn3
  192 MVA 18kV 3600 rpm2/RConn2 -- B/RConn1
  Va4/LConn1 -- 192 MVA 18kV 3600 rpm2/RConn1 -- A/RConn1

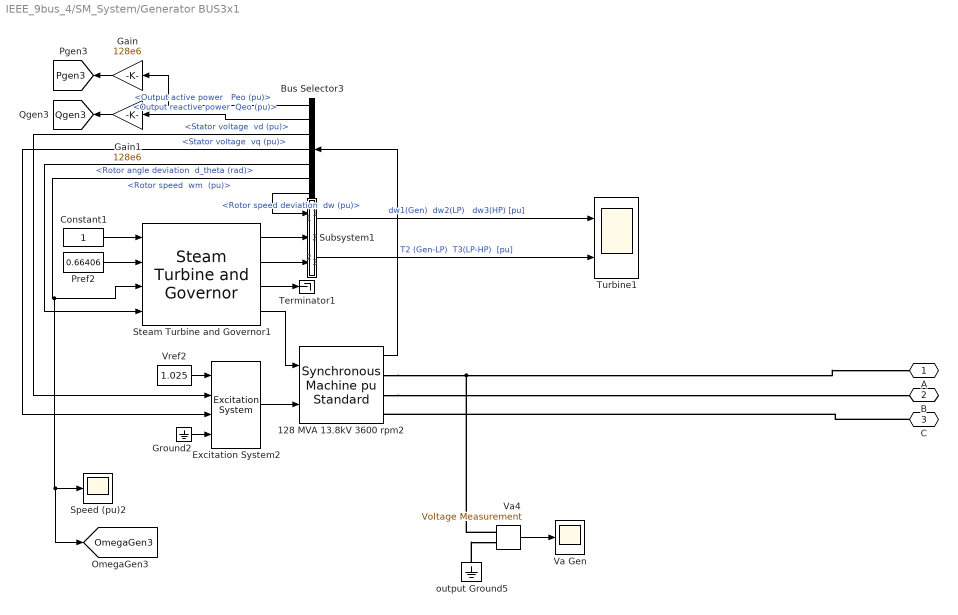
== system IEEE_9bus_4/SM_System/Generator BUS3x1 ==
  " Speed (pu)2" : Scope
      settings: TickLabels=on  TimeRange=150  YMin=0.99955  YMax=1  SaveName=Pm2
  128 MVA 13.8kV 3600 rpm2 : powerlib/Machines/Synchronous Machine pu Standard  PresetModel=No  MechanicalLoad=Mechanical power Pm  ShowDetailedParameters=on  RotorType=Round  Units=per unit standard parameters  MeasurementBus=off  NominalParameters="[ 128e6  13.8e3   60 ]"  Reactances1=[ 1.68, 0.232064, 0.1536, 1.609984, 0.32, 0.2176, 0.094976 ]  Reactances2="[ 1.305, 0.296, 0.252, 0.474,  0.243,  0.18 ]"  dAxisTimeConstants=Open-circuit  qAxisTimeConstants=Open-circuit  TimeConstants1="[ 4.4849  0.0681  0.1  ]"  TimeConstants2="[ 5.89, 0.05,  0.6, 0.05 ]"  TimeConstants3="[  4.49  0.0681  0.0513  ]"  TimeConstants4=[ 8.0, 0.03, 0.3371, 0.0295 ]  TimeConstants5=[ 1.01, 0.053, 0.1 ]  TimeConstants6=[ 1.3201, 0.023, 1.0, 0.07 ]  TimeConstants7="[  1.01  0.053  0.051266  ]"  TimeConstants8=[ 1.3201, 0.0231, 0.3371, 0.0295 ]  StatorResistance=0.000125  Mechanical="[ 3.01  0 1 ]"  PolePairs=1  InitialConditions=[0 -35.8791 0.653244 0.653244 0.653244 11.9635 -108.037 131.963 1.40212]  SetSaturation=off  Saturation=[0.6404,0.7127,0.8441,0.9214,0.9956,1.082,1.19,1.316,1.457;0.7,0.7698,0.8872,0.9466,0.9969,1.046,1.1,1.151,1.201]  LoadFlowParameters=[1 85000000 0 0 0]  TsPowergui=0  TsBlock=-1  IterativeModel=Trapezoidal non iterative  BusType=PV  Pref=85e6  Qref=0  Qmin=-Inf  Qmax=Inf  PLF=0  QLF=0
  Bus Selector3 : BusSelector  OutputSignals="Output active power   Peo (pu),Output reactive power  Qeo (pu),dq0 components.Stator voltage  vd (pu),dq0 components.Stator voltage  vq (pu),Mechanical.Rotor angle deviation  d_theta (rad),Mechanical.Rotor speed  wm  (pu),Mechanical.Rotor speed deviation  dw (pu)"
  Constant1 : Constant
  Excitation System2 : sps_avr/Excitation System  tr=20e-3  reg=[ 200, 0.02 ]  exc=[ 1, 0 ]  tgr=[ 12.0, 1.0 ]  damp=[ 0.03, 1.0 ]  sat=[ 0, 0 ]  lim=[ -10.0, 10.0, 0 ]  v0=[1.025 1.4021]
  Gain : Gain  Gain=128e6
  Gain1 : Gain  Gain=128e6
  Ground2 : Ground
  Pref2 : Constant  Value=0.66406
  Steam Turbine and Governor1 : powerlib/Machines/Steam Turbine and Governor  gentype=Tandem-compound (single mass)  reg1="[ 1  0.05    0 ]"  reg2="[ 0.001  0.1 ]"  reg3="[ -10.0 0.1   0.1 1.0 ]"  N=3600  turb1="[ 0.12  0.13  10.0   0.32   ]"  turb2="[ 0.48   0.25   0  0.27 ]"  HA="[  1.5498   0.24894  0  0 ]"  KA="[  83.47  42.702  0  0 ]"  DA="[  0.3104  0.05  0  0 ]*8"  ini1=0.66412  ini2=[1.88924e-008,-120.067]
  Subsystem1 : Subsystem
  Terminator1 : Terminator
  Turbine1 : Scope  NumInputPorts=2
      settings: TimeRange=0.5  YMin=-3e-07~-1  YMax=5e-08~1  SaveName=ScopeData2
  Va Gen : Scope
      settings: TickLabels=on  TimeRange=0.007300652369719236  YMin=-15000  YMax=15000  SaveName=vf4
  Va4 : powerlib/Measurements/Voltage Measurement  Tag=PoWeRsYsTeMmEaSuReMeNt  PhasorSimulation=off  OutputType=Magnitude  PSBequivalent=0
  Vref2 : Constant  Value=1.025
  output Ground5 : powerlib/Elements/Ground  LConnTagsString=a
  A : PMIOPort  Port=1  Side=Right
  B : PMIOPort  Port=2  Side=Right
  C : PMIOPort  Port=3  Side=Right
  tag scope: OmegaGen3=global, Pgen3=global, Qgen3=global
  wires:
  Constant1/1 -> Steam Turbine and Governor1/1
  Bus Selector3/5 -> Steam Turbine and Governor1/4  "<Rotor angle deviation  d_theta (rad)>"
  Subsystem1/2(T_23) -> Turbine1/2  "T2 (Gen-LP)  T3(LP-HP)  [pu]"
  Steam Turbine and Governor1/3 -> Terminator1/1
  Bus Selector3/7 -> Subsystem1/1(In1)  "<Rotor speed deviation  dw (pu)>"
  Vref2/1 -> Excitation System2/1
  Pref2/1 -> Steam Turbine and Governor1/2
  Steam Turbine and Governor1/1 -> Subsystem1/2(In2)
  Subsystem1/1(dw_123) -> Turbine1/1  "dw1(Gen)  dw2(LP)   dw3(HP) [pu]"
  Steam Turbine and Governor1/4 -> 128 MVA 13.8kV 3600 rpm2/1
  Steam Turbine and Governor1/2 -> Subsystem1/3(In3)
  Bus Selector3/6 -> [OmegaGen3], " Speed (pu)2"/1, Steam Turbine and Governor1/3  "<Rotor speed  wm  (pu)>"
  128 MVA 13.8kV 3600 rpm2/1 -> Bus Selector3/1
  Ground2/1 -> Excitation System2/4
  Bus Selector3/4 -> Excitation System2/3  "<Stator voltage  vq (pu)>"
  Bus Selector3/3 -> Excitation System2/2  "<Stator voltage  vd (pu)>"
  Excitation System2/1 -> 128 MVA 13.8kV 3600 rpm2/2
  Va4/1 -> Va Gen/1
  Gain/1 -> [Pgen3]
  Bus Selector3/1 -> Gain/1  "<Output active power   Peo (pu)>"
  Gain1/1 -> [Qgen3]
  Bus Selector3/2 -> Gain1/1  "<Output reactive power  Qeo (pu)>"
  connections:
  output Ground5/LConn1 -- Va4/LConn2
  C/RConn1 -- 128 MVA 13.8kV 3600 rpm2/RConn3
  128 MVA 13.8kV 3600 rpm2/RConn2 -- B/RConn1
  Va4/LConn1 -- 128 MVA 13.8kV 3600 rpm2/RConn1 -- A/RConn1

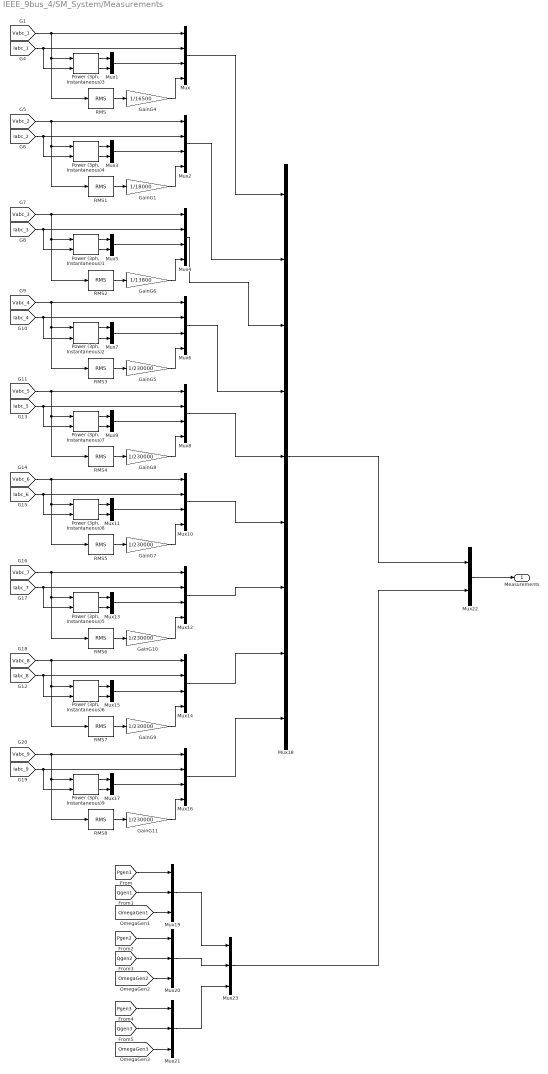
== system IEEE_9bus_4/SM_System/Measurements ==
  GainG1 : Gain  Gain=1/18000
  GainG{5,7..11} (6 alike) : Gain  Gain=1/230000
  GainG4 : Gain  Gain=1/16500
  GainG6 : Gain  Gain=1/13800
  Mux{,2,4,6,8,10,12,14,16} (9 alike) : Mux
  Mux{1,3,5,7,9,11,13,15,17,22} (10 alike) : Mux  Inputs=2
  Mux18 : Mux  Inputs=9
  Mux{19..21,23} (4 alike) : Mux  Inputs=3
  Power (3ph, Instantaneous){1..9} (9 alike) : powerlib_meascontrol/Measurements/Power (3ph, Instantaneous)
  RMS{,1..8} (9 alike) : powerlib_meascontrol/Measurements/RMS  TrueRMS=on  Freq=60  RMSInit=230  Ts=0
  Measurements : Outport
  wires:
  [Pgen2] -> Mux20/1
  [Qgen3] -> Mux21/2
  [Qgen2] -> Mux20/2
  [Qgen1] -> Mux19/2
  [Pgen1] -> Mux19/1
  [OmegaGen1] -> Mux19/3
  [Vabc_1] -> RMS/1, "Power (3ph, Instantaneous)3"/1, Mux/1
  RMS/1 -> GainG4/1
  [Iabc_1] -> "Power (3ph, Instantaneous)3"/2, Mux/2
  GainG4/1 -> Mux/4
  "Power (3ph, Instantaneous)3"/1 -> Mux1/1
  "Power (3ph, Instantaneous)3"/2 -> Mux1/2
  Mux1/1 -> Mux/3
  "Power (3ph, Instantaneous)4"/2 -> Mux3/2
  [Vabc_2] -> RMS1/1, "Power (3ph, Instantaneous)4"/1, Mux2/1
  [Iabc_2] -> "Power (3ph, Instantaneous)4"/2, Mux2/2
  "Power (3ph, Instantaneous)4"/1 -> Mux3/1
  RMS1/1 -> GainG1/1
  GainG1/1 -> Mux2/4
  Mux3/1 -> Mux2/3
  "Power (3ph, Instantaneous)1"/2 -> Mux5/2
  "Power (3ph, Instantaneous)2"/1 -> Mux7/1
  GainG5/1 -> Mux6/4
  [Iabc_4] -> "Power (3ph, Instantaneous)2"/2, Mux6/2
  RMS3/1 -> GainG5/1
  [Vabc_3] -> RMS2/1, "Power (3ph, Instantaneous)1"/1, Mux4/1
  [Vabc_4] -> RMS3/1, "Power (3ph, Instantaneous)2"/1, Mux6/1
  [Iabc_3] -> "Power (3ph, Instantaneous)1"/2, Mux4/2
  Mux7/1 -> Mux6/3
  "Power (3ph, Instantaneous)1"/1 -> Mux5/1
  RMS2/1 -> GainG6/1
  GainG6/1 -> Mux4/4
  Mux5/1 -> Mux4/3
  "Power (3ph, Instantaneous)2"/2 -> Mux7/2
  "Power (3ph, Instantaneous)7"/2 -> Mux9/2
  "Power (3ph, Instantaneous)8"/1 -> Mux11/1
  GainG7/1 -> Mux10/4
  [Iabc_6] -> "Power (3ph, Instantaneous)8"/2, Mux10/2
  RMS5/1 -> GainG7/1
  [Vabc_5] -> RMS4/1, "Power (3ph, Instantaneous)7"/1, Mux8/1
  [Vabc_6] -> RMS5/1, "Power (3ph, Instantaneous)8"/1, Mux10/1
  [Iabc_5] -> "Power (3ph, Instantaneous)7"/2, Mux8/2
  Mux11/1 -> Mux10/3
  "Power (3ph, Instantaneous)6"/2 -> Mux15/2
  Mux13/1 -> Mux12/3
  RMS6/1 -> GainG10/1
  GainG10/1 -> Mux12/4
  "Power (3ph, Instantaneous)5"/1 -> Mux13/1
  [Vabc_8] -> RMS7/1, "Power (3ph, Instantaneous)6"/1, Mux14/1
  [Iabc_7] -> "Power (3ph, Instantaneous)5"/2, Mux12/2
  [Vabc_7] -> RMS6/1, "Power (3ph, Instantaneous)5"/1, Mux12/1
  Mux15/1 -> Mux14/3
  "Power (3ph, Instantaneous)7"/1 -> Mux9/1
  [Iabc_8] -> "Power (3ph, Instantaneous)6"/2, Mux14/2
  RMS7/1 -> GainG9/1
  "Power (3ph, Instantaneous)6"/1 -> Mux15/1
  RMS4/1 -> GainG8/1
  "Power (3ph, Instantaneous)5"/2 -> Mux13/2
  GainG9/1 -> Mux14/4
  GainG8/1 -> Mux8/4
  Mux9/1 -> Mux8/3
  "Power (3ph, Instantaneous)8"/2 -> Mux11/2
  "Power (3ph, Instantaneous)9"/1 -> Mux17/1
  RMS8/1 -> GainG11/1
  [Iabc_9] -> "Power (3ph, Instantaneous)9"/2, Mux16/2
  "Power (3ph, Instantaneous)9"/2 -> Mux17/2
  GainG11/1 -> Mux16/4
  Mux17/1 -> Mux16/3
  [Vabc_9] -> RMS8/1, "Power (3ph, Instantaneous)9"/1, Mux16/1
  Mux/1 -> Mux18/1
  Mux2/1 -> Mux18/2
  Mux4/1 -> Mux18/3
  Mux6/1 -> Mux18/4
  Mux8/1 -> Mux18/5
  Mux10/1 -> Mux18/6
  Mux12/1 -> Mux18/7
  Mux14/1 -> Mux18/8
  Mux16/1 -> Mux18/9
  [OmegaGen2] -> Mux20/3
  [Pgen3] -> Mux21/1
  [OmegaGen3] -> Mux21/3
  Mux18/1 -> Mux22/1
  Mux23/1 -> Mux22/2
  Mux19/1 -> Mux23/1
  Mux20/1 -> Mux23/2
  Mux21/1 -> Mux23/3
  Mux22/1 -> Measurements/1

== system IEEE_9bus_4/SM_System/OPMonitor ==
  Mux8 : Mux  Inputs=3
  OpMonitor : rtlab/Monitoring/OpMonitor  compute_time=on  real_step=on  idle_time=off  nb_overruns=on  user_time=off  user_name=my_event_name,another_event_name
  Monitor : Outport
  wires:
  OpMonitor/1 -> Mux8/2
  OpMonitor/2 -> Mux8/3
  OpMonitor/3 -> Mux8/1
  Mux8/1 -> Monitor/1

== system IEEE_9bus_4/SM_System/Bus_4 230 KV/Three-Phase V-I Measurement1 ==
  Kv : Gain  Gain=Ki  SaturateOnIntegerOverflow=on  OutDataTypeStr=Inherit: Same as input  ParamDataTypeStr=Inherit: Same as input
  Kv1 : Gain  Gain=Kv  SaturateOnIntegerOverflow=on  OutDataTypeStr=Inherit: Same as input  ParamDataTypeStr=Inherit: Same as input
  Mode I : spsVIMeasurementModel/Complex
  Mode V : spsVIMeasurementModel/Complex
  Model : spsVIMeasurementModel/VI_phase  SystemSampleTime=-1
  A : PMIOPort  Port=1  Side=Left
  B : PMIOPort  Port=2  Side=Left
  C : PMIOPort  Port=3  Side=Left
  a : PMIOPort  Port=4  Side=Right
  b : PMIOPort  Port=5  Side=Right
  c : PMIOPort  Port=6  Side=Right
  tag scope: Iabc_4=global, Vabc_4=global
  wires:
  Model/2 -> Kv/1
  Model/1 -> Kv1/1
  Kv/1 -> Mode I/1
  Kv1/1 -> Mode V/1
  Mode I/1 -> [Iabc_4]
  Mode V/1 -> [Vabc_4]
  connections:
  Model/RConn3 -- c/RConn1
  Model/RConn1 -- a/RConn1
  Model/RConn2 -- b/RConn1
  Model/LConn3 -- C/RConn1
  Model/LConn1 -- A/RConn1
  Model/LConn2 -- B/RConn1

== system IEEE_9bus_4/SM_System/Bus_4 230 KV/Three-Phase V-I Measurement3 ==
  Kv : Gain  Gain=Ki  SaturateOnIntegerOverflow=on  OutDataTypeStr=Inherit: Same as input  ParamDataTypeStr=Inherit: Same as input
  Kv1 : Gain  Gain=Kv  SaturateOnIntegerOverflow=on  OutDataTypeStr=Inherit: Same as input  ParamDataTypeStr=Inherit: Same as input
  Mode I : spsVIMeasurementModel/Complex
  Mode V : spsVIMeasurementModel/Complex
  Model : spsVIMeasurementModel/VI_phase  SystemSampleTime=-1
  A : PMIOPort  Port=1  Side=Left
  B : PMIOPort  Port=2  Side=Left
  C : PMIOPort  Port=3  Side=Left
  a : PMIOPort  Port=4  Side=Right
  b : PMIOPort  Port=5  Side=Right
  c : PMIOPort  Port=6  Side=Right
  tag scope: Iabc_46=global, Vabc_46=global
  wires:
  Model/2 -> Kv/1
  Model/1 -> Kv1/1
  Kv/1 -> Mode I/1
  Kv1/1 -> Mode V/1
  Mode I/1 -> [Iabc_46]
  Mode V/1 -> [Vabc_46]
  connections:
  Model/RConn3 -- c/RConn1
  Model/RConn1 -- a/RConn1
  Model/RConn2 -- b/RConn1
  Model/LConn3 -- C/RConn1
  Model/LConn1 -- A/RConn1
  Model/LConn2 -- B/RConn1

== system IEEE_9bus_4/SM_System/Bus_7 230 KV/Three-Phase V-I Measurement1 ==
  Kv : Gain  Gain=Ki  SaturateOnIntegerOverflow=on  OutDataTypeStr=Inherit: Same as input  ParamDataTypeStr=Inherit: Same as input
  Kv1 : Gain  Gain=Kv  SaturateOnIntegerOverflow=on  OutDataTypeStr=Inherit: Same as input  ParamDataTypeStr=Inherit: Same as input
  Mode I : spsVIMeasurementModel/Complex
  Mode V : spsVIMeasurementModel/Complex
  Model : spsVIMeasurementModel/VI_phase  SystemSampleTime=-1
  A : PMIOPort  Port=1  Side=Left
  B : PMIOPort  Port=2  Side=Left
  C : PMIOPort  Port=3  Side=Left
  a : PMIOPort  Port=4  Side=Right
  b : PMIOPort  Port=5  Side=Right
  c : PMIOPort  Port=6  Side=Right
  tag scope: Iabc_7=global, Vabc_7=global
  wires:
  Model/2 -> Kv/1
  Model/1 -> Kv1/1
  Kv/1 -> Mode I/1
  Kv1/1 -> Mode V/1
  Mode I/1 -> [Iabc_7]
  Mode V/1 -> [Vabc_7]
  connections:
  Model/RConn3 -- c/RConn1
  Model/RConn1 -- a/RConn1
  Model/RConn2 -- b/RConn1
  Model/LConn3 -- C/RConn1
  Model/LConn1 -- A/RConn1
  Model/LConn2 -- B/RConn1

== system IEEE_9bus_4/SM_System/Bus_7 230 KV/Three-Phase V-I Measurement3 ==
  Kv : Gain  Gain=Ki  SaturateOnIntegerOverflow=on  OutDataTypeStr=Inherit: Same as input  ParamDataTypeStr=Inherit: Same as input
  Kv1 : Gain  Gain=Kv  SaturateOnIntegerOverflow=on  OutDataTypeStr=Inherit: Same as input  ParamDataTypeStr=Inherit: Same as input
  Mode I : spsVIMeasurementModel/Complex
  Mode V : spsVIMeasurementModel/Complex
  Model : spsVIMeasurementModel/VI_phase  SystemSampleTime=-1
  A : PMIOPort  Port=1  Side=Left
  B : PMIOPort  Port=2  Side=Left
  C : PMIOPort  Port=3  Side=Left
  a : PMIOPort  Port=4  Side=Right
  b : PMIOPort  Port=5  Side=Right
  c : PMIOPort  Port=6  Side=Right
  tag scope: Iab=global, Vabc=global
  wires:
  Model/2 -> Kv/1
  Model/1 -> Kv1/1
  Kv/1 -> Mode I/1
  Kv1/1 -> Mode V/1
  Mode I/1 -> [Iab]
  Mode V/1 -> [Vabc]
  connections:
  Model/RConn3 -- c/RConn1
  Model/RConn1 -- a/RConn1
  Model/RConn2 -- b/RConn1
  Model/LConn3 -- C/RConn1
  Model/LConn1 -- A/RConn1
  Model/LConn2 -- B/RConn1

== system IEEE_9bus_4/SM_System/Bus_9 230 KV/Three-Phase V-I Measurement1 ==
  Kv : Gain  Gain=Ki  SaturateOnIntegerOverflow=on  OutDataTypeStr=Inherit: Same as input  ParamDataTypeStr=Inherit: Same as input
  Kv1 : Gain  Gain=Kv  SaturateOnIntegerOverflow=on  OutDataTypeStr=Inherit: Same as input  ParamDataTypeStr=Inherit: Same as input
  Mode I : spsVIMeasurementModel/Complex
  Mode V : spsVIMeasurementModel/Complex
  Model : spsVIMeasurementModel/VI_phase  SystemSampleTime=-1
  A : PMIOPort  Port=1  Side=Left
  B : PMIOPort  Port=2  Side=Left
  C : PMIOPort  Port=3  Side=Left
  a : PMIOPort  Port=4  Side=Right
  b : PMIOPort  Port=5  Side=Right
  c : PMIOPort  Port=6  Side=Right
  tag scope: Iabc_9=global, Vabc_9=global
  wires:
  Model/2 -> Kv/1
  Model/1 -> Kv1/1
  Kv/1 -> Mode I/1
  Kv1/1 -> Mode V/1
  Mode I/1 -> [Iabc_9]
  Mode V/1 -> [Vabc_9]
  connections:
  Model/RConn3 -- c/RConn1
  Model/RConn1 -- a/RConn1
  Model/RConn2 -- b/RConn1
  Model/LConn3 -- C/RConn1
  Model/LConn1 -- A/RConn1
  Model/LConn2 -- B/RConn1

== system IEEE_9bus_4/SM_System/Bus_9 230 KV/Three-Phase V-I Measurement3 ==
  Kv : Gain  Gain=Ki  SaturateOnIntegerOverflow=on  OutDataTypeStr=Inherit: Same as input  ParamDataTypeStr=Inherit: Same as input
  Kv1 : Gain  Gain=Kv  SaturateOnIntegerOverflow=on  OutDataTypeStr=Inherit: Same as input  ParamDataTypeStr=Inherit: Same as input
  Mode I : spsVIMeasurementModel/Complex
  Mode V : spsVIMeasurementModel/Complex
  Model : spsVIMeasurementModel/VI_phase  SystemSampleTime=-1
  A : PMIOPort  Port=1  Side=Left
  B : PMIOPort  Port=2  Side=Left
  C : PMIOPort  Port=3  Side=Left
  a : PMIOPort  Port=4  Side=Right
  b : PMIOPort  Port=5  Side=Right
  c : PMIOPort  Port=6  Side=Right
  tag scope: Iabc=global, Vabc_10=global
  wires:
  Model/2 -> Kv/1
  Model/1 -> Kv1/1
  Kv/1 -> Mode I/1
  Kv1/1 -> Mode V/1
  Mode I/1 -> [Iabc]
  Mode V/1 -> [Vabc_10]
  connections:
  Model/RConn3 -- c/RConn1
  Model/RConn1 -- a/RConn1
  Model/RConn2 -- b/RConn1
  Model/LConn3 -- C/RConn1
  Model/LConn1 -- A/RConn1
  Model/LConn2 -- B/RConn1
